simulink model "FM_Modulation_Demodulation_03"  (R2021b)
settings: Solver=FixedStepDiscrete  StartTime=0.0  StopTime=10  RelTol=1e-3
undefined symbols (not defined in the file): DiscIntNeverNeededParam
libraries: commanapbnd3 x1, dsparch4 x1, commsynccomp2 x1
settings Model: Creator=Rajeev Ranjan  LastModifiedBy=Rajeev Ranjan

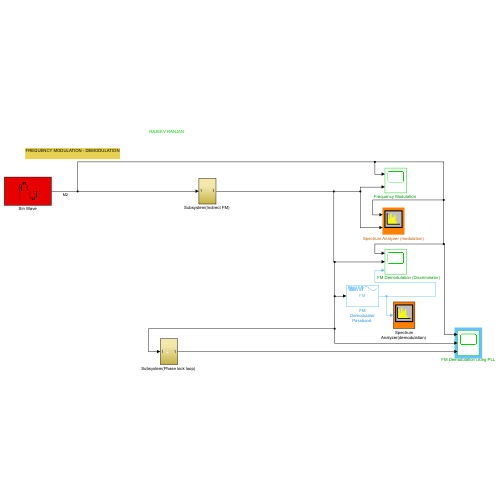
[thumbnail: Simulink's stored preview of the top-level diagram]
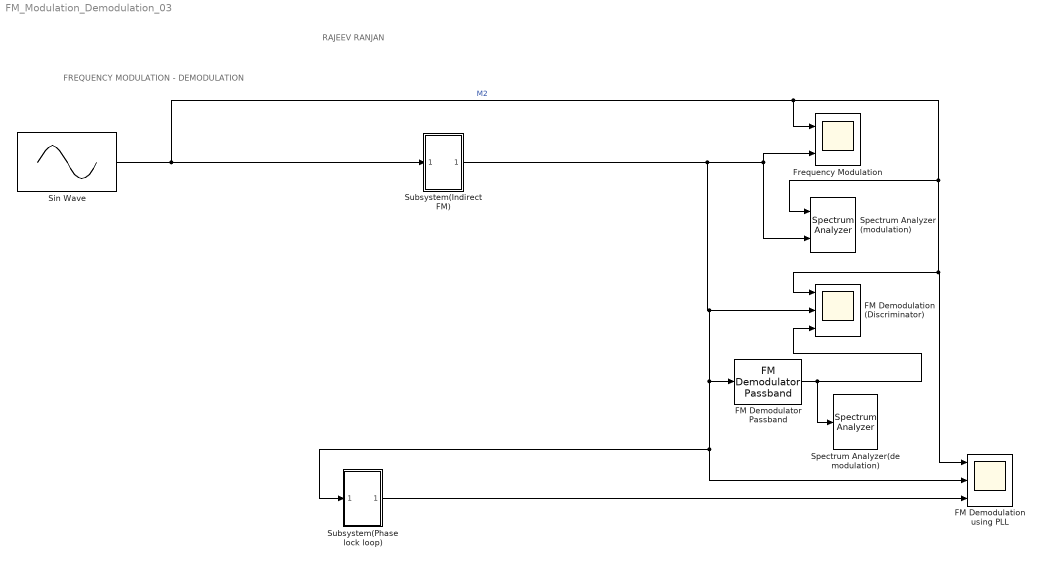
== system FM_Modulation_Demodulation_03 ==
  note: RAJEEV RANJAN
  note: FREQUENCY MODULATION - DEMODULATION
  "                       FM Demodulation (Discriminator) " : Scope  NumInputPorts=3
  "FM Demodulator Passband " : commanapbnd3/FM Demodulator Passband  Fc=20  Ph=0  Kc=10  Ho=200
      settings: SourceProductBaseCode=CM
  FM Demodulation using PLL : Scope  NumInputPorts=3
  "Frequency Modulation " : Scope  NumInputPorts=2
  Sin Wave : Sin  Frequency=4  SampleTime=1/1000
  "Spectrum Analyzer(demodulation) " : SpectrumAnalyzer
  Spectrum Analyzer (modulation) : SpectrumAnalyzer  NumInputPorts=2
  "Subsystem(Indirect FM) " : Subsystem
  "Subsystem(Phase lock loop) " : Subsystem
  wires:
  Sin Wave/1 -> "Subsystem(Indirect FM) "/1(In1), Spectrum Analyzer (modulation)/1, FM Demodulation using PLL/1, "                       FM Demodulation (Discriminator) "/1, "Frequency Modulation "/1  "M2"
  "FM Demodulator Passband "/1 -> "                       FM Demodulation (Discriminator) "/3, "Spectrum Analyzer(demodulation) "/1
  "Subsystem(Indirect FM) "/1(Out1) -> "Frequency Modulation "/2, Spectrum Analyzer (modulation)/2, "                       FM Demodulation (Discriminator) "/2, "FM Demodulator Passband "/1, FM Demodulation using PLL/2, "Subsystem(Phase lock loop) "/1(In1)
  "Subsystem(Phase lock loop) "/1(Out1) -> FM Demodulation using PLL/3

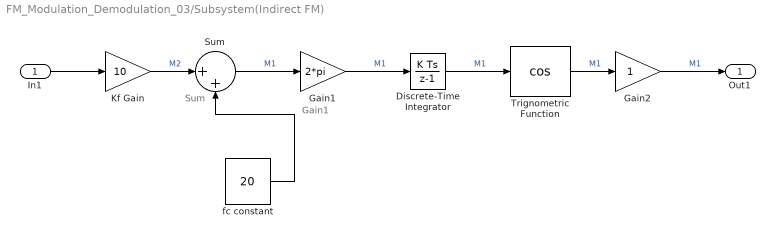
== system FM_Modulation_Demodulation_03/Subsystem(Indirect FM)  ==
  note: Sum
  note: Gain1
  In1 : Inport
  "Discrete-Time Integrator " : DiscreteIntegrator  SampleTime=-1  ICPrevOutput=DiscIntNeverNeededParam  ICPrevScaledInput=DiscIntNeverNeededParam
  Gain1 : Gain  Gain=2*pi
  "Gain2 " : Gain
  Kf Gain : Gain  Gain=10
  Sum : Sum  Inputs=|++
  Trignometric Function : Trigonometry  Operator=cos
  fc constant : Constant  Value=20
  Out1 : Outport
  wires:
  Gain1/1 -> "Discrete-Time Integrator "/1  "M1"
  Sum/1 -> Gain1/1  "M1"
  Kf Gain/1 -> Sum/1  "M2"
  "Gain2 "/1 -> Out1/1  "M1"
  In1/1 -> Kf Gain/1
  "Discrete-Time Integrator "/1 -> Trignometric Function/1  "M1"
  Trignometric Function/1 -> "Gain2 "/1  "M1"
  fc constant/1 -> Sum/2

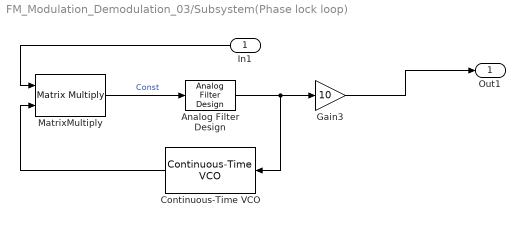
== system FM_Modulation_Demodulation_03/Subsystem(Phase lock loop)  ==
  In1 : Inport
  "Analog Filter Design " : dsparch4/Analog Filter Design  method=Butterworth  filttype=Lowpass  N=10  Wlo=2  Whi=80  Rp=2  Rs=40
  "Continuous-Time VCO " : commsynccomp2/Continuous-Time VCO  Ac=1  Fc=20  Kc=10/(2*pi)  Ph=pi/2
      settings: SourceProductBaseCode=CM
  "Gain3 " : Gain  Gain=10
  MatrixMultiply : Product  Multiplication=Matrix(*)
  Out1 : Outport
  wires:
  "Analog Filter Design "/1 -> "Continuous-Time VCO "/1, "Gain3 "/1
  "Continuous-Time VCO "/1 -> MatrixMultiply/2
  In1/1 -> MatrixMultiply/1
  MatrixMultiply/1 -> "Analog Filter Design "/1  "Const"
  "Gain3 "/1 -> Out1/1
